simulink model "main"  (R2022a)
settings: Solver=FixedStepDiscrete  StartTime=0.0  StopTime=Inf  FixedStep=(50e-6)-(sim_en*4.995e-5)  RelTol=1e-3  EnableMultiTasking=on
model workspace (MAT data in the model file):
  Param : Simulink.Parameter (value not decoded)
  ac_ok : Simulink.Signal (value not decoded)
  ac_ok_120 : Simulink.Signal (value not decoded)
  bulk_voltage : Simulink.Signal (value not decoded)
  burstduty_integ_max : Simulink.Signal (value not decoded)
  burstduty_integ_min : Simulink.Signal (value not decoded)
  burstduty_ki : Simulink.Signal (value not decoded)
  burstduty_kp : Simulink.Signal (value not decoded)
  calib_ok : Simulink.Signal (value not decoded)
  can_addr1 : Simulink.Signal (value not decoded)
  can_addr2 : Simulink.Signal (value not decoded)
  can_addr3 : Simulink.Signal (value not decoded)
  can_addr4 : Simulink.Signal (value not decoded)
  can_data_rx : Simulink.Signal (value not decoded)
  can_data_tx : Simulink.Signal (value not decoded)
  can_timeout_120 : Simulink.Signal (value not decoded)
  chksum_scircv : Simulink.Signal (value not decoded)
  clllc_en_120 : Simulink.Signal (value not decoded)
  clllc_fault_120 : Simulink.Signal (value not decoded)
  clllc_ok_120 : Simulink.Signal (value not decoded)
  cmpss1h : Simulink.Signal (value not decoded)
  cmpss1l : Simulink.Signal (value not decoded)
  cmpss2h : Simulink.Signal (value not decoded)
  cmpss2l : Simulink.Signal (value not decoded)
  cmpss3h : Simulink.Signal (value not decoded)
  cmpss3l : Simulink.Signal (value not decoded)
  cmpss4h : Simulink.Signal (value not decoded)
  cmpss4l : Simulink.Signal (value not decoded)
  cmpss5h : Simulink.Signal (value not decoded)
  cmpss5l : Simulink.Signal (value not decoded)
  cmpss6h : Simulink.Signal (value not decoded)
  cmpss6l : Simulink.Signal (value not decoded)
  cmpss7h : Simulink.Signal (value not decoded)
  cmpss7l : Simulink.Signal (value not decoded)
  cmpss8h : Simulink.Signal (value not decoded)
  cmpss8l : Simulink.Signal (value not decoded)
  cnt_idle : Simulink.Signal (value not decoded)
  cnt_orps : Simulink.Signal (value not decoded)
  cnt_scircv : Simulink.Signal (value not decoded)
  cnt_scixmt : Simulink.Signal (value not decoded)
  cnt_scixmt_func : Simulink.Signal (value not decoded)
  cnt_temp_mux : Simulink.Signal (value not decoded)
  cnt_vdroop : Simulink.Signal (value not decoded)
  config_ok : Simulink.Signal (value not decoded)
  control_en : Simulink.Signal (value not decoded)
  cp_ready_120 : Simulink.Signal (value not decoded)
  d2d_en : Simulink.Signal (value not decoded)
  dchg_off : Simulink.Signal (value not decoded)
  debug_dacb : Simulink.Signal (value not decoded)
  debug_dacc : Simulink.Signal (value not decoded)
  debug_msg1 : Simulink.Signal (value not decoded)
  debug_msg2 : Simulink.Signal (value not decoded)
  debug_msg3 : Simulink.Signal (value not decoded)
  debug_msg4 : Simulink.Signal (value not decoded)
  debug_msg5 : Simulink.Signal (value not decoded)
  debug_msg6 : Simulink.Signal (value not decoded)
  dir_v2g : Simulink.Signal (value not decoded)
  eoss_llc1 : Simulink.Signal (value not decoded)
  eoss_llc2 : Simulink.Signal (value not decoded)
  eoss_orps : Simulink.Signal (value not decoded)
  fault_ocp : Simulink.Signal (value not decoded)
  fault_otp : Simulink.Signal (value not decoded)
  fault_ovp : Simulink.Signal (value not decoded)
  fut_en : Simulink.Signal (value not decoded)
  fwd_en_120 : Simulink.Signal (value not decoded)
  gain_llc1_sec_idc : Simulink.Signal (value not decoded)
  gain_llc1_temp_sr : Simulink.Signal (value not decoded)
  gain_llc2_sec_idc : Simulink.Signal (value not decoded)
  gain_vbat : Simulink.Signal (value not decoded)
  gain_vbulk : Simulink.Signal (value not decoded)
  gain_vout : Simulink.Signal (value not decoded)
  input_current_phasea : Simulink.Signal (value not decoded)
  input_current_phaseb : Simulink.Signal (value not decoded)
  input_current_phasec : Simulink.Signal (value not decoded)
  input_freq : Simulink.Signal (value not decoded)
  input_power : Simulink.Signal (value not decoded)
  input_voltage_phasea : Simulink.Signal (value not decoded)
  input_voltage_phaseb : Simulink.Signal (value not decoded)
  input_voltage_phasec : Simulink.Signal (value not decoded)
  ishare_arbiter : Simulink.Signal (value not decoded)
  ishare_thresh : Simulink.Signal (value not decoded)
  led_g : Simulink.Signal (value not decoded)
  led_r : Simulink.Signal (value not decoded)
  led_y : Simulink.Signal (value not decoded)
  llc1_burst_integ : Simulink.Signal (value not decoded)
  llc1_burstduty_buffer : Simulink.Signal (value not decoded)
  llc1_pfm_error : Simulink.Signal (value not decoded)
  llc1_pfm_integ : Simulink.Signal (value not decoded)
  llc1_pfm_prop : Simulink.Signal (value not decoded)
  llc1_pri_idc : Simulink.Signal (value not decoded)
  llc1_ps_buffer : Simulink.Signal (value not decoded)
  llc1_pspwm_error : Simulink.Signal (value not decoded)
  llc1_pspwm_integ : Simulink.Signal (value not decoded)
  llc1_pspwm_prop : Simulink.Signal (value not decoded)
  llc1_sec_idc : Simulink.Signal (value not decoded)
  llc1_temp_sr : Simulink.Signal (value not decoded)
  llc1_ts_tbctr_buffer : Simulink.Signal (value not decoded)
  llc2_burst_integ : Simulink.Signal (value not decoded)
  llc2_burstduty_buffer : Simulink.Signal (value not decoded)
  llc2_en : Simulink.Signal (value not decoded)
  llc2_en_buffer : Simulink.Signal (value not decoded)
  llc2_pfm_error : Simulink.Signal (value not decoded)
  llc2_pfm_integ : Simulink.Signal (value not decoded)
  llc2_pfm_prop : Simulink.Signal (value not decoded)
  llc2_pri_idc : Simulink.Signal (value not decoded)
  llc2_ps_buffer : Simulink.Signal (value not decoded)
  llc2_pspwm_error : Simulink.Signal (value not decoded)
  llc2_pspwm_integ : Simulink.Signal (value not decoded)
  llc2_pspwm_prop : Simulink.Signal (value not decoded)
  llc2_sec_idc : Simulink.Signal (value not decoded)
  llc2_temp_sr : Simulink.Signal (value not decoded)
  llc2_ts_tbctr_buffer : Simulink.Signal (value not decoded)
  loop_adcint : Simulink.Signal (value not decoded)
  loop_control : Simulink.Signal (value not decoded)
  loop_idle : Simulink.Signal (value not decoded)
  mid_bulk_voltage : Simulink.Signal (value not decoded)
  mode_120 : Simulink.Signal (value not decoded)
  mode_cc_cv : Simulink.Signal (value not decoded)
  myParam : mpt.Parameter (value not decoded)
  obc_ok_120 : Simulink.Signal (value not decoded)
  offset_llc1_sec_idc : Simulink.Signal (value not decoded)
  offset_llc1_temp_sr : Simulink.Signal (value not decoded)
  offset_llc2_sec_idc : Simulink.Signal (value not decoded)
  offset_vbat : Simulink.Signal (value not decoded)
  offset_vbulk : Simulink.Signal (value not decoded)
  offset_vout : Simulink.Signal (value not decoded)
  openloop_en : Simulink.Signal (value not decoded)
  openloop_fault_en : Simulink.Signal (value not decoded)
  ot_fault_120 : Simulink.Signal (value not decoded)
  pfc_en : Simulink.Signal (value not decoded)
  pfc_en_120 : Simulink.Signal (value not decoded)
  pfc_fw_revision : Simulink.Signal (value not decoded)
  pfc_fw_revision_bootloader : Simulink.Signal (value not decoded)
  pfc_fw_revision_debug : Simulink.Signal (value not decoded)
  pfc_ok : Simulink.Signal (value not decoded)
  pfc_ok_120 : Simulink.Signal (value not decoded)
  pfm_a0 : Simulink.Signal (value not decoded)
  pfm_a1 : Simulink.Signal (value not decoded)
  pfm_integ_max : Simulink.Signal (value not decoded)
  pfm_integ_min : Simulink.Signal (value not decoded)
  pfm_ki : Simulink.Signal (value not decoded)
  pfm_kp : Simulink.Signal (value not decoded)
  pri_fut_en : Simulink.Signal (value not decoded)
  pri_fut_en_buffer : Simulink.Signal (value not decoded)
  pri_halfbridge_en : Simulink.Signal (value not decoded)
  pri_halfbridge_en_buffer : Simulink.Signal (value not decoded)
  pspwm_integ_max : Simulink.Signal (value not decoded)
  pspwm_integ_min : Simulink.Signal (value not decoded)
  pspwm_ki : Simulink.Signal (value not decoded)
  pspwm_kp : Simulink.Signal (value not decoded)
  ref_idclink_max : Simulink.Signal (value not decoded)
  ref_iout : Simulink.Signal (value not decoded)
  ref_iout_calib : Simulink.Signal (value not decoded)
  ref_iout_llc1 : Simulink.Signal (value not decoded)
  ref_iout_llc1_calib : Simulink.Signal (value not decoded)
  ref_iout_llc2 : Simulink.Signal (value not decoded)
  ref_iout_llc2_calib : Simulink.Signal (value not decoded)
  ref_pout : Simulink.Signal (value not decoded)
  ref_ss_llc1 : Simulink.Signal (value not decoded)
  ref_ss_llc2 : Simulink.Signal (value not decoded)
  ref_ss_orps : Simulink.Signal (value not decoded)
  ref_vbat : Simulink.Signal (value not decoded)
  ref_vbat_calib : Simulink.Signal (value not decoded)
  ref_vbulk : Simulink.Signal (value not decoded)
  ref_vbulk_calib : Simulink.Signal (value not decoded)
  ref_vbulk_llc1_calib : Simulink.Signal (value not decoded)
  ref_vbulk_llc2_calib : Simulink.Signal (value not decoded)
  ref_vout : Simulink.Signal (value not decoded)
  ref_vout_calib : Simulink.Signal (value not decoded)
  relay_en : Simulink.Signal (value not decoded)
  reset_flag : Simulink.Signal (value not decoded)
  rev_en_120 : Simulink.Signal (value not decoded)
  runtime_control : Simulink.Signal (value not decoded)
  runtime_idle : Simulink.Signal (value not decoded)
  scircv_buffer : Simulink.Signal (value not decoded)
  scircv_buffer_tmp : Simulink.Signal (value not decoded)
  scircv_buffer_tmp_idx0 : Simulink.Signal (value not decoded)
  scircv_chksum : Simulink.Signal (value not decoded)
  scircv_chksum_ok : Simulink.Signal (value not decoded)
  scircv_parse_ok : Simulink.Signal (value not decoded)
  scixmt_buffer : Simulink.Signal (value not decoded)
  scixmt_chksum : Simulink.Signal (value not decoded)
  scixmt_func : Simulink.Signal (value not decoded)
  scixmt_word0_lsb : Simulink.Signal (value not decoded)
  scixmt_word0_msb : Simulink.Signal (value not decoded)
  scixmt_word1_lsb : Simulink.Signal (value not decoded)
  scixmt_word1_msb : Simulink.Signal (value not decoded)
  scixmt_word2_lsb : Simulink.Signal (value not decoded)
  scixmt_word2_msb : Simulink.Signal (value not decoded)
  scixmt_wr : Simulink.Signal (value not decoded)
  ss_step : Simulink.Signal (value not decoded)
  state_calib : Simulink.Signal (value not decoded)
  state_control : Simulink.Signal (value not decoded)
  state_hkeep : Simulink.Signal (value not decoded)
  status_cmpss : Simulink.Signal (value not decoded)
  status_control : Simulink.Signal (value not decoded)
  status_digin : Simulink.Signal (value not decoded)
  status_digout : Simulink.Signal (value not decoded)
  status_fault : Simulink.Signal (value not decoded)
  status_input : Simulink.Signal (value not decoded)
  status_pfc : Simulink.Signal (value not decoded)
  temp_inlet : Simulink.Signal (value not decoded)
  temp_llc1_fet_hs : Simulink.Signal (value not decoded)
  temp_llc2_fet_hs : Simulink.Signal (value not decoded)
  temp_mux : Simulink.Signal (value not decoded)
  temp_mux_s0 : Simulink.Signal (value not decoded)
  temp_mux_s1 : Simulink.Signal (value not decoded)
  temp_mux_s2 : Simulink.Signal (value not decoded)
  temp_outlet : Simulink.Signal (value not decoded)
  temp_pfc_fet_hsa : Simulink.Signal (value not decoded)
  temp_pfc_fet_hsb : Simulink.Signal (value not decoded)
  temp_pfc_fet_hsc : Simulink.Signal (value not decoded)
  temp_pfc_fet_lsa : Simulink.Signal (value not decoded)
  temp_pfc_fet_lsb : Simulink.Signal (value not decoded)
  temp_pfc_fet_lsc : Simulink.Signal (value not decoded)
  test_mode : Simulink.Signal (value not decoded)
  tfcv_cc : Simulink.Signal (value not decoded)
  tfcv_cc_llc2 : Simulink.Signal (value not decoded)
  tfcv_cv : Simulink.Signal (value not decoded)
  tfcv_sr_en : Simulink.Signal (value not decoded)
  tfv_assert_llc1_pri_idc : Simulink.Signal (value not decoded)
  tfv_assert_llc1_sec_idc : Simulink.Signal (value not decoded)
  tfv_assert_llc1_temp_sr : Simulink.Signal (value not decoded)
  tfv_assert_llc2_pri_idc : Simulink.Signal (value not decoded)
  tfv_assert_llc2_sec_idc : Simulink.Signal (value not decoded)
  tfv_assert_llc2_temp_sr : Simulink.Signal (value not decoded)
  tfv_assert_temp_outlet : Simulink.Signal (value not decoded)
  tfv_assert_vaux_uv : Simulink.Signal (value not decoded)
  tfv_assert_vbat : Simulink.Signal (value not decoded)
  tfv_assert_vbulk : Simulink.Signal (value not decoded)
  tfv_assert_vout : Simulink.Signal (value not decoded)
  tfv_cnt_tz : Simulink.Signal (value not decoded)
  tfv_deassert_llc1_pri_idc : Simulink.Signal (value not decoded)
  tfv_deassert_llc1_sec_idc : Simulink.Signal (value not decoded)
  tfv_deassert_llc1_temp_sr : Simulink.Signal (value not decoded)
  tfv_deassert_llc2_pri_idc : Simulink.Signal (value not decoded)
  tfv_deassert_llc2_sec_idc : Simulink.Signal (value not decoded)
  tfv_deassert_llc2_temp_sr : Simulink.Signal (value not decoded)
  tfv_deassert_temp_outlet : Simulink.Signal (value not decoded)
  tfv_deassert_vaux_uv : Simulink.Signal (value not decoded)
  tfv_deassert_vbat : Simulink.Signal (value not decoded)
  tfv_deassert_vbulk : Simulink.Signal (value not decoded)
  tfv_deassert_vout : Simulink.Signal (value not decoded)
  tfv_llc1_pri_idc : Simulink.Signal (value not decoded)
  tfv_llc1_sec_idc : Simulink.Signal (value not decoded)
  tfv_llc1_temp_sr : Simulink.Signal (value not decoded)
  tfv_llc2_pri_idc : Simulink.Signal (value not decoded)
  tfv_llc2_sec_idc : Simulink.Signal (value not decoded)
  tfv_llc2_temp_sr : Simulink.Signal (value not decoded)
  tfv_temp_outlet : Simulink.Signal (value not decoded)
  tfv_vaux_uv : Simulink.Signal (value not decoded)
  tfv_vbat : Simulink.Signal (value not decoded)
  tfv_vbulk : Simulink.Signal (value not decoded)
  tfv_vout : Simulink.Signal (value not decoded)
  timer_1ms : Simulink.Signal (value not decoded)
  tz : Simulink.Signal (value not decoded)
  valve_en : Simulink.Signal (value not decoded)
  vaux : Simulink.Signal (value not decoded)
  vbat : Simulink.Signal (value not decoded)
  vbulk : Simulink.Signal (value not decoded)
  vout : Simulink.Signal (value not decoded)
undefined symbols (not defined in the file or in its folder): CAN_O_INT, CANA_BASE, Down, GPTRIP1SEL, GPTRIP2SEL, TZ1, TZ2, Up
libraries: hdlsllib x159, simulink x94, c2802xlib x32, c2837xDlib x19, c2807xlib x16, c280xlib x13, canmsglib x8, idelinklib_common x2, c2000lib x1, c281xlib x1
(part 16 of 20)

== system main/Task_Manager/init/codegen/init/tztl_clb/clb ==
  note: // Enabling EPWM1 to enable CLB1
      | SysCtl_enablePeripheral(SYSCTL_PERIPH_CLK_EPWM1);
      | CLB_enableCLB(CLB1_BASE);
      | initTILE0(CLB1_BASE);
      |
      | // Enabling EPWM2 to enable CLB2
      | SysCtl_enablePeripheral(SYSCTL_PERIPH_CLK_EPWM1);
      | CLB_enableCLB(CLB2_BASE);
      | initTILE1(CLB2_BASE);
      |
      |
      |
      | // Select Global input instead of local input for all CLB IN
      | CLB_configLocalInputMux(CLB1_BASE, CLB_IN0, CLB_LOCAL_IN_MUX_GLOBAL_IN);
      | CLB_configLocalInputMux(CLB1_BASE, CLB_IN1, CLB_LOCAL_IN_MUX_GLOBAL_IN);
      | CLB_configLocalInputMux(CLB1_BASE, CLB_IN2, CLB_LOCAL_IN_MUX_GLOBAL_IN);
      | CLB_configLocalInputMux(CLB1_BASE, CLB_IN3, CLB_LOCAL_IN_MUX_GLOBAL_IN);
      | CLB_configLocalInputMux(CLB1_BASE, CLB_IN4, CLB_LOCAL_IN_MUX_GLOBAL_IN);
      | CLB_configLocalInputMux(CLB1_BASE, CLB_IN5, CLB_LOCAL_IN_MUX_GLOBAL_IN);
      | CLB_configLocalInputMux(CLB1_BASE, CLB_IN6, CLB_LOCAL_IN_MUX_GLOBAL_IN);
      | CLB_configLocalInputMux(CLB1_BASE, CLB_IN7, CLB_LOCAL_IN_MUX_GLOBAL_IN);
      |
      | CLB_configLocalInputMux(CLB2_BASE, CLB_IN0, CLB_LOCAL_IN_MUX_GLOBAL_IN);
      | CLB_configLocalInputMux(CLB2_BASE, CLB_IN1, CLB_LOCAL_IN_MUX_GLOBAL_IN);
      | CLB_configLocalInputMux(CLB2_BASE, CLB_IN2, CLB_LOCAL_IN_MUX_GLOBAL_IN);
      | CLB_configLocalInputMux(CLB2_BASE, CLB_IN3, CLB_LOCAL_IN_MUX_GLOBAL_IN);
      | CLB_configLocalInputMux(CLB2_BASE, CLB_IN4, CLB_LOCAL_IN_MUX_GLOBAL_IN);
      | CLB_configLocalInputMux(CLB2_BASE, CLB_IN5, CLB_LOCAL_IN_MUX_GLOBAL_IN);
      | CLB_configLocalInputMux(CLB2_BASE, CLB_IN6, CLB_LOCAL_IN_MUX_GLOBAL_IN);
      | CLB_configLocalInputMux(CLB2_BASE, CLB_IN7, CLB_LOCAL_IN_MUX_GLOBAL_IN);
      |
      |
      | // Select AUXSIG for CLBx, IN0/1/2
      | CLB_configGlobalInputMux(CLB1_BASE, CLB_IN0, CLB_GLOBAL_IN_MUX_CLB_AUXSIG0);
      | CLB_configGlobalInputMux(CLB1_BASE, CLB_IN1, CLB_GLOBAL_IN_MUX_CLB_AUXSIG1);
      | CLB_configGlobalInputMux(CLB1_BASE, CLB_IN2, CLB_GLOBAL_IN_MUX_EPWM1_CTR_PRD);
      | CLB_configGlobalInputMux(CLB2_BASE, CLB_IN0, CLB_GLOBAL_IN_MUX_CLB_AUXSIG2);
      | CLB_configGlobalInputMux(CLB2_BASE, CLB_IN1, CLB_GLOBAL_IN_MUX_CLB_AUXSIG3);
      | CLB_configGlobalInputMux(CLB2_BASE, CLB_IN2, CLB_GLOBAL_IN_MUX_EPWM1_CTR_ZERO);
      |
      |
      | // Unused inputs below
      | CLB_configGlobalInputMux(CLB1_BASE, CLB_IN3, CLB_GLOBAL_IN_MUX_EPWM1A);
      | CLB_configGlobalInputMux(CLB1_BASE, CLB_IN4, CLB_GLOBAL_IN_MUX_EPWM1A);
      | CLB_configGlobalInputMux(CLB1_BASE, CLB_IN5, CLB_GLOBAL_IN_MUX_EPWM1A);
      | CLB_configGlobalInputMux(CLB1_BASE, CLB_IN6, CLB_GLOBAL_IN_MUX_EPWM1A);
      | CLB_configGlobalInputMux(CLB1_BASE, CLB_IN7, CLB_GLOBAL_IN_MUX_EPWM1A);
      | CLB_configGlobalInputMux(CLB2_BASE, CLB_IN3, CLB_GLOBAL_IN_MUX_EPWM1A);
      | CLB_configGlobalInputMux(CLB2_BASE, CLB_IN4, CLB_GLOBAL_IN_MUX_EPWM1A);
      | CLB_configGlobalInputMux(CLB2_BASE, CLB_IN5, CLB_GLOBAL_IN_MUX_EPWM1A);
      | CLB_configGlobalInputMux(CLB2_BASE, CLB_IN6, CLB_GLOBAL_IN_MUX_EPWM1A);
      | CLB_configGlobalInputMux(CLB2_BASE, CLB_IN7, CLB_GLOBAL_IN_MUX_EPWM1A);
      |
      |
      | // Set CLB_IN to mux external
      | CLB_configGPInputMux(CLB1_BASE, CLB_IN0, CLB_GP_IN_MUX_EXTERNAL);
      | CLB_configGPInputMux(CLB1_BASE, CLB_IN1, CLB_GP_IN_MUX_EXTERNAL);
      | CLB_configGPInputMux(CLB1_BASE, CLB_IN2, CLB_GP_IN_MUX_EXTERNAL);
      | CLB_configGPInputMux(CLB2_BASE, CLB_IN0, CLB_GP_IN_MUX_EXTERNAL);
      | CLB_configGPInputMux(CLB2_BASE, CLB_IN1, CLB_GP_IN_MUX_EXTERNAL);
      | CLB_configGPInputMux(CLB2_BASE, CLB_IN2, CLB_GP_IN_MUX_EXTERNAL);
      |
      |
      | // Set unused inputs to GP register
      | CLB_configGPInputMux(CLB1_BASE, CLB_IN3, CLB_GP_IN_MUX_GP_REG);
      | CLB_configGPInputMux(CLB1_BASE, CLB_IN4, CLB_GP_IN_MUX_GP_REG);
      | CLB_configGPInputMux(CLB1_BASE, CLB_IN5, CLB_GP_IN_MUX_GP_REG);
      | CLB_configGPInputMux(CLB1_BASE, CLB_IN6, CLB_GP_IN_MUX_GP_REG);
      | CLB_configGPInputMux(CLB1_BASE, CLB_IN7, CLB_GP_IN_MUX_GP_REG);
      | CLB_configGPInputMux(CLB2_BASE, CLB_IN3, CLB_GP_IN_MUX_GP_REG);
      | CLB_configGPInputMux(CLB2_BASE, CLB_IN4, CLB_GP_IN_MUX_GP_REG);
      | CLB_configGPInputMux(CLB2_BASE, CLB_IN5, CLB_GP_IN_MUX_GP_REG);
      | CLB_configGPInputMux(CLB2_BASE, CLB_IN6, CLB_GP_IN_MUX_GP_REG);
      | CLB_configGPInputMux(CLB2_BASE, CLB_IN7, CLB_GP_IN_MUX_GP_REG);
      |
      |
      | // Configure CLB-XBAR AUXSIG
      | XBAR_setCLBMuxConfig(XBAR_AUXSIG0, XBAR_CLB_MUX08_CMPSS5_CTRIPH);
      | XBAR_enableCLBMux(XBAR_AUXSIG0, XBAR_MUX08);
      | XBAR_setCLBMuxConfig(XBAR_AUXSIG1, XBAR_CLB_MUX09_CMPSS5_CTRIPL);
      | XBAR_enableCLBMux(XBAR_AUXSIG1, XBAR_MUX09);
      | XBAR_setCLBMuxConfig(XBAR_AUXSIG2, XBAR_CLB_MUX10_CMPSS6_CTRIPH);
      | XBAR_enableCLBMux(XBAR_AUXSIG2, XBAR_MUX10);
      | XBAR_setCLBMuxConfig(XBAR_AUXSIG3, XBAR_CLB_MUX11_CMPSS6_CTRIPL);
      | XBAR_enableCLBMux(XBAR_AUXSIG3, XBAR_MUX11);
      |
      |
      |
      | // Configure ePWM XBAR
      | XBAR_setEPWMMuxConfig(XBAR_TRIP9, XBAR_EPWM_MUX01_CLB1_OUT4);
      | XBAR_enableEPWMMux(XBAR_TRIP9, XBAR_MUX01);
      | XBAR_setEPWMMuxConfig(XBAR_TRIP10, XBAR_EPWM_MUX05_CLB2_OUT4);
      | XBAR_enableEPWMMux(XBAR_TRIP10, XBAR_MUX05);
  function : TriggerPort  TriggerType=function-call  VariantControl=Variant
  System Initialize : Subsystem  mask(System Initialize){ShowInLibBrowser=0}
      mask prompts: ShowInLibBrowser "Simulink:masks:CustCodeMaskParam1_MP"
      settings: CopyFcn=cccopyfcn(gcb)  OpenFcn=ccopenfcn('System Initialize Function')
      mask Help: eval('feval(''rtwprivate'',''rtwhelpview'',''rtw_sys_initialize_block'')');
      mask Display: disp('System\nInitialize');

== system main/Task_Manager/init/codegen/init/tztl_clb/tzctl ==
  note: //TZCTL configures TZ action of a DCxEVTy event
      | //0b00=HI-Z, 0b01=HI, 0b10=LO, 0b11=DN
      | EALLOW;
      |
      | //LLC1_PRI_PS
      | EPwm1Regs.TZCTL.bit.DCAEVT1 = 0b11; //Do nothing
      | EPwm1Regs.TZCTL.bit.DCAEVT2 = 0b11; //Do nothing
      | EPwm1Regs.TZCTL.bit.DCBEVT1 = 0b11; //Do nothing
      | EPwm1Regs.TZCTL.bit.DCBEVT2 = 0b11; //Do nothing
      |
      | //LLC1_PRI_STD
      | EPwm2Regs.TZCTL.bit.DCAEVT1 = 0b11; //Do nothing
      | EPwm2Regs.TZCTL.bit.DCAEVT2 = 0b11; //Do nothing
      | EPwm2Regs.TZCTL.bit.DCBEVT1 = 0b11; //Do nothing
      | EPwm2Regs.TZCTL.bit.DCBEVT2 = 0b11; //Do nothing
      |
      | //LLC1_SEC_PS
      | EPwm7Regs.TZCTL.bit.DCAEVT1 = 0b10; //LO
      | EPwm7Regs.TZCTL.bit.DCAEVT2 = 0b01; //HI
      | EPwm7Regs.TZCTL.bit.DCBEVT1 = 0b10; //LO
      | EPwm7Regs.TZCTL.bit.DCBEVT2 = 0b01; //HI
      |
      | //LLC1_SEC_STD
      | EPwm8Regs.TZCTL.bit.DCAEVT1 = 0b10; //LO
      | EPwm8Regs.TZCTL.bit.DCAEVT2 = 0b01; //HI
      | EPwm8Regs.TZCTL.bit.DCBEVT1 = 0b10; //LO
      | EPwm8Regs.TZCTL.bit.DCBEVT2 = 0b01; //HI
      |
      | EDIS;
  function : TriggerPort  TriggerType=function-call  VariantControl=Variant
  System Initialize : Subsystem  mask(System Initialize){ShowInLibBrowser=0}
      mask prompts: ShowInLibBrowser "Simulink:masks:CustCodeMaskParam1_MP"
      settings: CopyFcn=cccopyfcn(gcb)  OpenFcn=ccopenfcn('System Initialize Function')
      mask Help: eval('feval(''rtwprivate'',''rtwhelpview'',''rtw_sys_initialize_block'')');
      mask Display: disp('System\nInitialize');

== system main/interrupt_adca/burst_control/burst/disPulse/Variant Subsystem/codegen/g2v_prifullbridge ==
  note: EPwm1Regs.AQCSFRC.bit.CSFA = 0b1; //force low
      | EPwm1Regs.AQCSFRC.bit.CSFB = 0b1; //force low
      | EPwm2Regs.AQCSFRC.bit.CSFA = 0b1; //force low
      | EPwm2Regs.AQCSFRC.bit.CSFB = 0b1; //force low
      |
      | EPwm7Regs.AQCSFRC.bit.CSFA = 0b1; //force low
      | EPwm7Regs.AQCSFRC.bit.CSFB = 0b1; //force low
      | EPwm8Regs.AQCSFRC.bit.CSFA = 0b1; //force low
      | EPwm8Regs.AQCSFRC.bit.CSFB = 0b1; //force low
  Action Port : ActionPort  ActionPortLabel=if((u1==0))
  System Outputs1 : Subsystem  mask(System Outputs){ShowInLibBrowser=0}
      mask prompts: ShowInLibBrowser "Simulink:masks:CustCodeMaskParam1_MP"
      settings: CopyFcn=cccopyfcn(gcb)  OpenFcn=ccopenfcn('System Outputs Function')
      mask Help: eval('feval(''rtwprivate'',''rtwhelpview'',''rtw_sys_outputs_block'')');
      mask DialogControl ShowInLibBrowser Prompt: Mask Parameter 1:
      mask Display: disp('System\nOutputs');

== system main/interrupt_adca/burst_control/burst/disPulse/Variant Subsystem/codegen/v2g_prifullbridge ==
  note: EPwm1Regs.AQCSFRC.bit.CSFA = 0b1; //force low
      | EPwm1Regs.AQCSFRC.bit.CSFB = 0b1; //force low
      | EPwm2Regs.AQCSFRC.bit.CSFA = 0b1; //force low
      | EPwm2Regs.AQCSFRC.bit.CSFB = 0b1; //force low
      | EPwm7Regs.AQCSFRC.bit.CSFA = 0b1; //force low
      | EPwm7Regs.AQCSFRC.bit.CSFB = 0b1; //force low
      | EPwm8Regs.AQCSFRC.bit.CSFA = 0b1; //force low
      | EPwm8Regs.AQCSFRC.bit.CSFB = 0b1; //force low
  Action Port : ActionPort  ActionPortLabel=elseif((u1==1))
  System Outputs1 : Subsystem  mask(System Outputs){ShowInLibBrowser=0}
      mask prompts: ShowInLibBrowser "Simulink:masks:CustCodeMaskParam1_MP"
      settings: CopyFcn=cccopyfcn(gcb)  OpenFcn=ccopenfcn('System Outputs Function')
      mask Help: eval('feval(''rtwprivate'',''rtwhelpview'',''rtw_sys_outputs_block'')');
      mask DialogControl ShowInLibBrowser Prompt: Mask Parameter 1:
      mask Display: disp('System\nOutputs');

== system main/interrupt_adca/burst_control/burst/disPulse/Variant Subsystem/sim/g2v_prifullbridge ==
  note: EPwm1Regs.AQCSFRC.bit.CSFA = 0b1; //force low
      | EPwm1Regs.AQCSFRC.bit.CSFB = 0b1; //force low
      | EPwm2Regs.AQCSFRC.bit.CSFA = 0b1; //force low
      | EPwm2Regs.AQCSFRC.bit.CSFB = 0b1; //force low
      | EPwm7Regs.AQCSFRC.bit.CSFA = 0b0; //force disable
      | EPwm7Regs.AQCSFRC.bit.CSFB = 0b0; //force disable
      | EPwm8Regs.AQCSFRC.bit.CSFA = 0b0; //force disable
      | EPwm8Regs.AQCSFRC.bit.CSFB = 0b0; //force disable
  note: LLC1 SEC
  note: LLC1 PRI
  Action Port : ActionPort
  Constant{,1,4..5} (4 alike) : Constant  OutDataTypeStr=boolean
  Constant{2..3,6..7} (4 alike) : Constant  Value=0  OutDataTypeStr=boolean
  Data Store Write : DataStoreWrite  DataStoreName=epwm1_aqcsfrc_csfa  IndexOptions=Index vector (dialog)  Indices=1  OutputSizes=1
  Data Store Write1 : DataStoreWrite  DataStoreName=epwm1_aqcsfrc_csfb  IndexOptions=Index vector (dialog)  Indices=1  OutputSizes=1
  Data Store Write2 : DataStoreWrite  DataStoreName=epwm7_aqcsfrc_csfa  IndexOptions=Index vector (dialog)  Indices=1  OutputSizes=1
  Data Store Write3 : DataStoreWrite  DataStoreName=epwm7_aqcsfrc_csfb  IndexOptions=Index vector (dialog)  Indices=1  OutputSizes=1
  Data Store Write4 : DataStoreWrite  DataStoreName=epwm2_aqcsfrc_csfa  IndexOptions=Index vector (dialog)  Indices=1  OutputSizes=1
  Data Store Write5 : DataStoreWrite  DataStoreName=epwm2_aqcsfrc_csfb  IndexOptions=Index vector (dialog)  Indices=1  OutputSizes=1
  Data Store Write6 : DataStoreWrite  DataStoreName=epwm8_aqcsfrc_csfa  IndexOptions=Index vector (dialog)  Indices=1  OutputSizes=1
  Data Store Write7 : DataStoreWrite  DataStoreName=epwm8_aqcsfrc_csfb  IndexOptions=Index vector (dialog)  Indices=1  OutputSizes=1
  wires:
  Constant3/1 -> Data Store Write3/1
  Constant2/1 -> Data Store Write2/1
  Constant6/1 -> Data Store Write6/1
  Constant/1 -> Data Store Write/1
  Constant4/1 -> Data Store Write4/1
  Constant1/1 -> Data Store Write1/1
  Constant5/1 -> Data Store Write5/1
  Constant7/1 -> Data Store Write7/1

== system main/interrupt_adca/burst_control/burst/disPulse/Variant Subsystem/sim/v2g_prifullbridge ==
  note: EPwm1Regs.AQCSFRC.bit.CSFA = 0b0; //force disabled
      | EPwm1Regs.AQCSFRC.bit.CSFB = 0b0; //force disabled
      | EPwm2Regs.AQCSFRC.bit.CSFA = 0b0; //force disabled
      | EPwm2Regs.AQCSFRC.bit.CSFB = 0b0; //force disabled
      | EPwm7Regs.AQCSFRC.bit.CSFA = 0b1; //force low
      | EPwm7Regs.AQCSFRC.bit.CSFB = 0b1; //force low
      | EPwm8Regs.AQCSFRC.bit.CSFA = 0b1; //force low
      | EPwm8Regs.AQCSFRC.bit.CSFB = 0b1; //force low
  note: LLC1 SEC
  note: LLC1 PRI
  Action Port : ActionPort
  Constant{,1,4..5} (4 alike) : Constant  Value=0  OutDataTypeStr=boolean
  Constant{2..3,6..7} (4 alike) : Constant  OutDataTypeStr=boolean
  Data Store Write : DataStoreWrite  DataStoreName=epwm1_aqcsfrc_csfa  IndexOptions=Index vector (dialog)  Indices=1  OutputSizes=1
  Data Store Write1 : DataStoreWrite  DataStoreName=epwm1_aqcsfrc_csfb  IndexOptions=Index vector (dialog)  Indices=1  OutputSizes=1
  Data Store Write2 : DataStoreWrite  DataStoreName=epwm7_aqcsfrc_csfa  IndexOptions=Index vector (dialog)  Indices=1  OutputSizes=1
  Data Store Write3 : DataStoreWrite  DataStoreName=epwm7_aqcsfrc_csfb  IndexOptions=Index vector (dialog)  Indices=1  OutputSizes=1
  Data Store Write4 : DataStoreWrite  DataStoreName=epwm2_aqcsfrc_csfa  IndexOptions=Index vector (dialog)  Indices=1  OutputSizes=1
  Data Store Write5 : DataStoreWrite  DataStoreName=epwm2_aqcsfrc_csfb  IndexOptions=Index vector (dialog)  Indices=1  OutputSizes=1
  Data Store Write6 : DataStoreWrite  DataStoreName=epwm8_aqcsfrc_csfa  IndexOptions=Index vector (dialog)  Indices=1  OutputSizes=1
  Data Store Write7 : DataStoreWrite  DataStoreName=epwm8_aqcsfrc_csfb  IndexOptions=Index vector (dialog)  Indices=1  OutputSizes=1
  wires:
  Constant6/1 -> Data Store Write6/1
  Constant2/1 -> Data Store Write2/1
  Constant3/1 -> Data Store Write3/1
  Constant5/1 -> Data Store Write5/1
  Constant1/1 -> Data Store Write1/1
  Constant4/1 -> Data Store Write4/1
  Constant/1 -> Data Store Write/1
  Constant7/1 -> Data Store Write7/1

== system main/interrupt_adca/burst_control/burst/disPwm/disPwm/codegen/System Outputs1 ==

== system main/interrupt_adca/burst_control/burst/enPulse/enPwm/codegen/System Outputs ==

== system main/Control_State_Machine/control/configSr/configXbarEpwmtrip/codegen/g2v_prifullbridge/clb/System Outputs1 ==

== system main/Control_State_Machine/control/configSr/configXbarEpwmtrip/codegen/g2v_prifullbridge/tzctl/System Outputs ==

== system main/Control_State_Machine/control/configSr/configXbarEpwmtrip/codegen/v2g_prifullbridge/clb/System Outputs3 ==

== system main/Control_State_Machine/control/configSr/configXbarEpwmtrip/codegen/v2g_prifullbridge/tzctl/System Outputs1 ==

== system main/Task_Manager/Tmr_20mS/codegen/Task_20mS/Rx_Handler/ProcessMB10/Mode_Cmd ==
  Input : Inport
  Action Port : ActionPort  ActionPortLabel=if(u1 == 1)
  Data Store Write1 : DataStoreWrite  DataStoreName=u8ModeCmd  IndexOptions=Index vector (dialog)  Indices=1  OutputSizes=1
  wires:
  Input/1 -> Data Store Write1/1

== system main/Task_Manager/Tmr_20mS/codegen/Task_20mS/Rx_Handler/ProcessMB11/Red_Mode_Cmd ==
  Input : Inport
  Action Port : ActionPort  ActionPortLabel=if(u1 == 1)
  Data Store Write1 : DataStoreWrite  DataStoreName=u8RedunModeCmd  IndexOptions=Index vector (dialog)  Indices=1  OutputSizes=1
  wires:
  Input/1 -> Data Store Write1/1

== system main/Task_Manager/Tmr_20mS/codegen/Task_20mS/Rx_Handler/ProcessMB12/Debug_Cmd ==
  Action Port : ActionPort  ActionPortLabel=elseif( u1==2)
  Constant3 : Constant  Value=[1:1]
  Data Store Read1 : DataStoreRead  DataStoreName=u8CanDataRx12  IndexOptions=Index vector (dialog)  Indices=1  OutputSizes=1
  Debug En/Dis : Subsystem  TreatAsAtomicUnit=on
  If1 : If  IfExpression=u1 == hex2dec('0xDA')  ElseIfExpressions=u1 == hex2dec('0xDB')
  Open Loop En Dis : Subsystem  TreatAsAtomicUnit=on
  Selector3 : Selector  IndexMode=Zero-based  InputPortWidth=8  IndexOptions=Index vector (port)  Indices=[1 3]  OutputSizes=1
  wires:
  Selector3/1 -> If1/1
  Constant3/1 -> Selector3/2
  Data Store Read1/1 -> Selector3/1
  If1/1 -> Debug En/Dis/Action
  If1/2 -> Open Loop En Dis/Action

== system main/Task_Manager/Tmr_20mS/codegen/Task_20mS/Rx_Handler/ProcessMB12/Debug_Read ==
  Action Port : ActionPort  ActionPortLabel=if(u1 == 0)
  Constant2 : Constant  Value=[1:1]
  Data Store Read : DataStoreRead  DataStoreName=u8CanDataRx12  IndexOptions=Index vector (dialog)  Indices=1  OutputSizes=1
  Debug_Cmd : Subsystem  TreatAsAtomicUnit=on
  Equal{,1..3} (4 alike) : RelationalOperator  Operator===  OutDataTypeStr=boolean  RndMeth=Simplest  InputSameDT=off
  If : If  IfExpression=u1 == 1
  OR : Logic  Operator=OR  Inputs=4  IconShape=distinctive  AllPortsSameDT=off  OutDataTypeStr=boolean
  RdReq_Calib : Constant  Value=0xD0
  RdReq_Deb1 : Constant  Value=0xD1
  RdReq_Deb2 : Constant  Value=0xD2
  RdReq_FwRev : Constant  Value=0xF0
  Selector1 : Selector  IndexMode=Zero-based  InputPortWidth=8  IndexOptions=Index vector (port)  Indices=[1 3]  OutputSizes=1
  wires:
  Constant2/1 -> Selector1/2
  Data Store Read/1 -> Selector1/1
  RdReq_FwRev/1 -> Equal/2
  RdReq_Calib/1 -> Equal1/2
  Selector1/1 -> Equal1/1, Equal2/1, Debug_Cmd/1(Input), Equal3/1, Equal/1
  RdReq_Deb2/1 -> Equal3/2
  RdReq_Deb1/1 -> Equal2/2
  Equal2/1 -> OR/3
  Equal3/1 -> OR/4
  Equal1/1 -> OR/2
  Equal/1 -> OR/1
  OR/1 -> If/1
  If/1 -> Debug_Cmd/Action

== system main/Task_Manager/Tmr_20mS/codegen/Task_20mS/Rx_Handler/ProcessMB12/Debug_Write ==
  Action Port : ActionPort  ActionPortLabel=elseif(u1 ==1)

== system main/Task_Manager/Tmr_20mS/codegen/Task_20mS/Tx_Handler/Run Tx Routine/TxReadRequest ==
  Action Port : ActionPort  ActionPortLabel=if(u1 == 1 & u2 == 1)
  Constant1 : Constant  Value=0  OutDataTypeStr=boolean
  Data Store Read2 : DataStoreRead  DataStoreName=u8RdReqMsgPntr  IndexOptions=Index vector (dialog)  Indices=1  OutputSizes=1
  Data Store Write1 : DataStoreWrite  DataStoreName=b01_ReadRequest  IndexOptions=Index vector (dialog)  Indices=1  OutputSizes=1
  Switch Case : SwitchCase  CaseConditions={0xF0, 0xD0, 0xD1, 0xD2}  ShowDefaultCase=off
  Tx Cal Data ID145 : Subsystem  TreatAsAtomicUnit=on
  Tx FW Rev ID144 : Subsystem  TreatAsAtomicUnit=on
  Tx TxDeb Dat1 146 : Subsystem  TreatAsAtomicUnit=on
  Tx TxDeb Dat2 147 : Subsystem  TreatAsAtomicUnit=on
  wires:
  Data Store Read2/1 -> Switch Case/1
  Switch Case/1 -> Tx FW Rev ID144/Action
  Switch Case/2 -> Tx Cal Data ID145/Action
  Switch Case/3 -> Tx TxDeb Dat1 146/Action
  Switch Case/4 -> Tx TxDeb Dat2 147/Action
  Constant1/1 -> Data Store Write1/1

== system main/Task_Manager/Tmr_20mS/codegen/Task_20mS/Tx_Handler/Run Tx Routine/TxStatusData ==
  Action Port : ActionPort  ActionPortLabel=else
  Data Store Read2 : DataStoreRead  DataStoreName=u8CanTxIndex  IndexOptions=Index vector (dialog)  Indices=1  OutputSizes=1
  Switch Case : SwitchCase  CaseConditions={0, 1, 2, 3, 4}  ShowDefaultCase=off
  Tx Sec Status ID120 : Subsystem  TreatAsAtomicUnit=on
  Tx Sec1 ID140 : Subsystem  TreatAsAtomicUnit=on
  Tx Sec2 ID141 : Subsystem  TreatAsAtomicUnit=on
  Tx Sec3 ID142 : Subsystem  TreatAsAtomicUnit=on
  Tx Sec4 ID143 : Subsystem  TreatAsAtomicUnit=on
  wires:
  Data Store Read2/1 -> Switch Case/1
  Switch Case/1 -> Tx Sec Status ID120/Action
  Switch Case/2 -> Tx Sec1 ID140/Action
  Switch Case/3 -> Tx Sec2 ID141/Action
  Switch Case/4 -> Tx Sec3 ID142/Action
  Switch Case/5 -> Tx Sec4 ID143/Action

== system main/Task_Manager/idle/idle_task/comm_npc/comm_npc/COMM_NPC.calcScixmtChksum/calc_chksum/For Iterator Subsystem ==
  scixmt_buffer : Inport
  Bitwise XOR : simulink/Logic and Bit Operations/Bitwise Operator  logicop=XOR  UseBitMask=off  NumInputPorts=2  BitMask=bin2dec('11011001')  BitMaskRealWorld=Stored Integer
  Data Store Read1 : DataStoreRead  DataStoreName=scixmt_chksum  IndexOptions=Index vector (dialog)  Indices=1  OutputSizes=1
  Data Store Write : DataStoreWrite  DataStoreName=scixmt_chksum  IndexOptions=Index vector (dialog)  Indices=1  OutputSizes=1
  For Iterator : ForIterator  IterationLimit=9  IndexMode=Zero-based  IterationVariableDataType=uint8
  Selector : Selector  IndexMode=Zero-based  InputPortWidth=12  IndexOptions=Index vector (port)  Indices=[1 3]  OutputSizes=1
  wires:
  For Iterator/1 -> Selector/2
  scixmt_buffer/1 -> Selector/1
  Selector/1 -> Bitwise XOR/1
  Bitwise XOR/1 -> Data Store Write/1
  Data Store Read1/1 -> Bitwise XOR/2

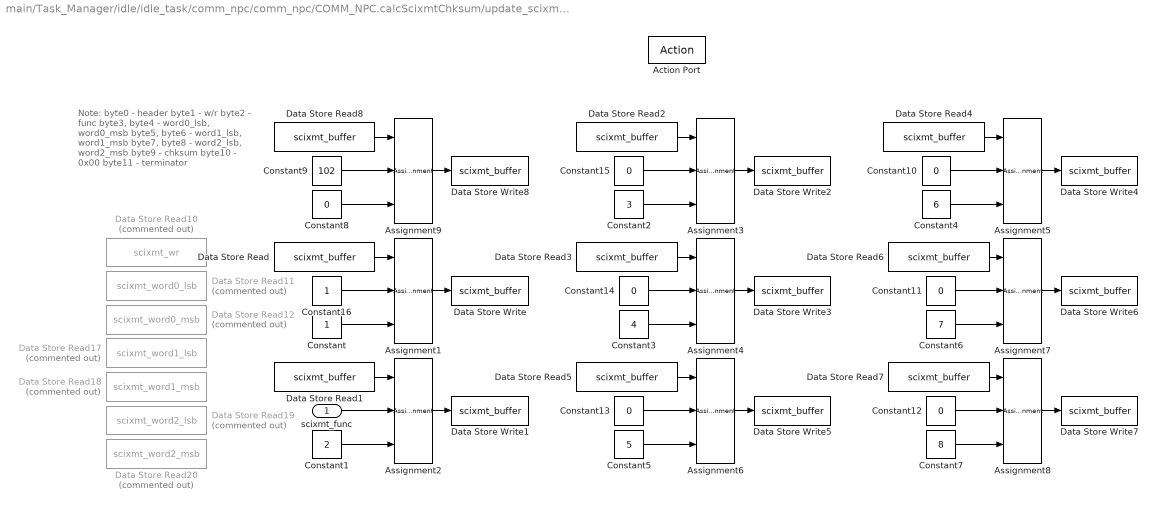
== system main/Task_Manager/idle/idle_task/comm_npc/comm_npc/COMM_NPC.calcScixmtChksum/update_scixmt_buffer/default ==
  note: Note:
      | byte0 - header
      | byte1 - w/r
      | byte2 - func
      | byte3, byte4 - word0_lsb, word0_msb
      | byte5, byte6 - word1_lsb, word1_msb
      | byte7, byte8 - word2_lsb, word2_msb
      | byte9 - chksum
      | byte10 - 0x00
      | byte11 - terminator
  scixmt_func : Inport
  Action Port : ActionPort  ActionPortLabel=else
  Assignment{1..9} (9 alike) : Assignment  IndexMode=Zero-based  DiagnosticForDimensions=Warning  IndexOptions=Index vector (port)  Indices=1  OutputSizes=1
  Constant : Constant  OutDataTypeStr=uint8
  Constant1 : Constant  Value=2  OutDataTypeStr=uint8
  Constant{8,10..15} (7 alike) : Constant  Value=0  OutDataTypeStr=uint8
  Constant16 : Constant  OutDataTypeStr=uint8
  Constant2 : Constant  Value=3  OutDataTypeStr=uint8
  Constant3 : Constant  Value=4  OutDataTypeStr=uint8
  Constant4 : Constant  Value=6  OutDataTypeStr=uint8
  Constant5 : Constant  Value=5  OutDataTypeStr=uint8
  Constant6 : Constant  Value=7  OutDataTypeStr=uint8
  Constant7 : Constant  Value=8  OutDataTypeStr=uint8
  Constant9 : Constant  Value=102  OutDataTypeStr=uint8
  Data Store Read{,1..8} (9 alike) : DataStoreRead  DataStoreName=scixmt_buffer  IndexOptions=Index vector (dialog)  Indices=1  OutputSizes=1
  Data Store Read10 : DataStoreRead  Commented=on  DataStoreName=scixmt_wr  IndexOptions=Index vector (dialog)  Indices=1  OutputSizes=1
  Data Store Read11 : DataStoreRead  Commented=on  DataStoreName=scixmt_word0_lsb  IndexOptions=Index vector (dialog)  Indices=1  OutputSizes=1
  Data Store Read12 : DataStoreRead  Commented=on  DataStoreName=scixmt_word0_msb  IndexOptions=Index vector (dialog)  Indices=1  OutputSizes=1
  Data Store Read17 : DataStoreRead  Commented=on  DataStoreName=scixmt_word1_lsb  IndexOptions=Index vector (dialog)  Indices=1  OutputSizes=1
  Data Store Read18 : DataStoreRead  Commented=on  DataStoreName=scixmt_word1_msb  IndexOptions=Index vector (dialog)  Indices=1  OutputSizes=1
  Data Store Read19 : DataStoreRead  Commented=on  DataStoreName=scixmt_word2_lsb  IndexOptions=Index vector (dialog)  Indices=1  OutputSizes=1
  Data Store Read20 : DataStoreRead  Commented=on  DataStoreName=scixmt_word2_msb  IndexOptions=Index vector (dialog)  Indices=1  OutputSizes=1
  Data Store Write{,1..8} (9 alike) : DataStoreWrite  DataStoreName=scixmt_buffer  IndexOptions=Index vector (dialog)  Indices=1  OutputSizes=1
  wires:
  scixmt_func/1 -> Assignment2/2
  Constant13/1 -> Assignment6/2
  Assignment1/1 -> Data Store Write/1
  Constant9/1 -> Assignment9/2
  Data Store Read8/1 -> Assignment9/1
  Assignment5/1 -> Data Store Write4/1
  Assignment9/1 -> Data Store Write8/1
  Constant11/1 -> Assignment7/2
  Constant/1 -> Assignment1/3
  Assignment6/1 -> Data Store Write5/1
  Constant2/1 -> Assignment3/3
  Constant5/1 -> Assignment6/3
  Data Store Read5/1 -> Assignment6/1
  Data Store Read7/1 -> Assignment8/1
  Constant4/1 -> Assignment5/3
  Data Store Read6/1 -> Assignment7/1
  Constant6/1 -> Assignment7/3
  Data Store Read1/1 -> Assignment2/1
  Assignment7/1 -> Data Store Write6/1
  Data Store Read4/1 -> Assignment5/1
  Constant7/1 -> Assignment8/3
  Data Store Read3/1 -> Assignment4/1
  Assignment8/1 -> Data Store Write7/1
  Data Store Read2/1 -> Assignment3/1
  Constant12/1 -> Assignment8/2
  Data Store Read/1 -> Assignment1/1
  Constant3/1 -> Assignment4/3
  Assignment3/1 -> Data Store Write2/1
  Constant10/1 -> Assignment5/2
  Constant14/1 -> Assignment4/2
  Assignment4/1 -> Data Store Write3/1
  Constant15/1 -> Assignment3/2
  Constant1/1 -> Assignment2/3
  Constant8/1 -> Assignment9/3
  Assignment2/1 -> Data Store Write1/1
  Constant16/1 -> Assignment1/2

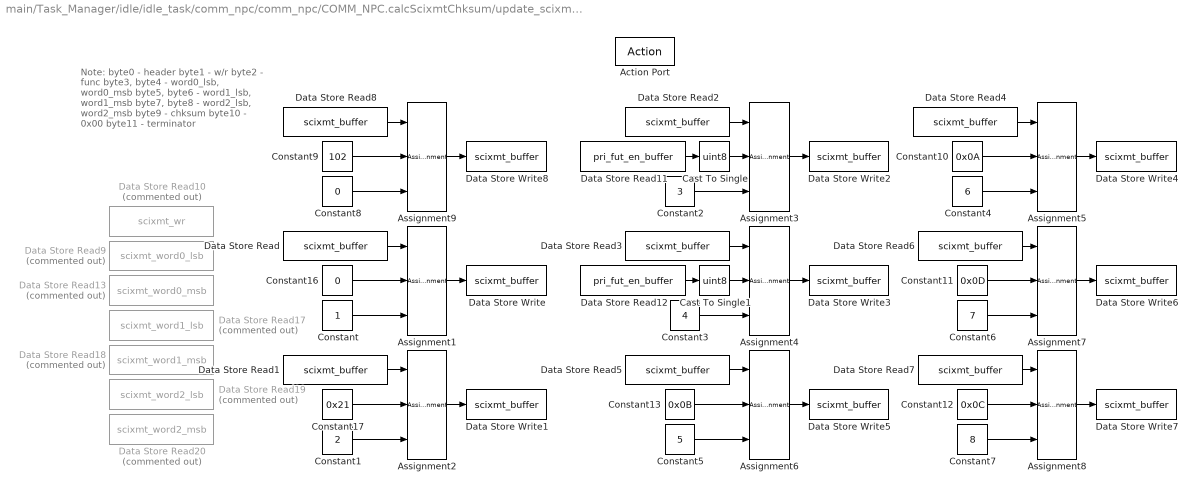
== system main/Task_Manager/idle/idle_task/comm_npc/comm_npc/COMM_NPC.calcScixmtChksum/update_scixmt_buffer/pri_fut_en ==
  note: Note:
      | byte0 - header
      | byte1 - w/r
      | byte2 - func
      | byte3, byte4 - word0_lsb, word0_msb
      | byte5, byte6 - word1_lsb, word1_msb
      | byte7, byte8 - word2_lsb, word2_msb
      | byte9 - chksum
      | byte10 - 0x00
      | byte11 - terminator
  Action Port : ActionPort  ActionPortLabel=if(u1 == 33)
  Assignment{1..9} (9 alike) : Assignment  IndexMode=Zero-based  DiagnosticForDimensions=Warning  IndexOptions=Index vector (port)  Indices=1  OutputSizes=1
  Cast To Single : DataTypeConversion  OutDataTypeStr=uint8  SaturateOnIntegerOverflow=off  RndMeth=Floor
  Cast To Single1 : DataTypeConversion  OutDataTypeStr=uint8  SaturateOnIntegerOverflow=off  RndMeth=Floor
  Constant : Constant  OutDataTypeStr=uint8
  Constant1 : Constant  Value=2  OutDataTypeStr=uint8
  Constant10 : Constant  Value=0x0A  OutDataTypeStr=uint8
  Constant11 : Constant  Value=0x0D  OutDataTypeStr=uint8
  Constant12 : Constant  Value=0x0C  OutDataTypeStr=uint8
  Constant13 : Constant  Value=0x0B  OutDataTypeStr=uint8
  Constant16 : Constant  Value=0  OutDataTypeStr=uint8
  Constant17 : Constant  Value=0x21  OutDataTypeStr=uint8
  Constant2 : Constant  Value=3  OutDataTypeStr=uint8
  Constant3 : Constant  Value=4  OutDataTypeStr=uint8
  Constant4 : Constant  Value=6  OutDataTypeStr=uint8
  Constant5 : Constant  Value=5  OutDataTypeStr=uint8
  Constant6 : Constant  Value=7  OutDataTypeStr=uint8
  Constant7 : Constant  Value=8  OutDataTypeStr=uint8
  Constant8 : Constant  Value=0  OutDataTypeStr=uint8
  Constant9 : Constant  Value=102  OutDataTypeStr=uint8
  Data Store Read{,1..8} (9 alike) : DataStoreRead  DataStoreName=scixmt_buffer  IndexOptions=Index vector (dialog)  Indices=1  OutputSizes=1
  Data Store Read10 : DataStoreRead  Commented=on  DataStoreName=scixmt_wr  IndexOptions=Index vector (dialog)  Indices=1  OutputSizes=1
  Data Store Read11 : DataStoreRead  DataStoreName=pri_fut_en_buffer  IndexOptions=Index vector (dialog)  Indices=1  OutputSizes=1
  Data Store Read12 : DataStoreRead  DataStoreName=pri_fut_en_buffer  IndexOptions=Index vector (dialog)  Indices=1  OutputSizes=1
  Data Store Read13 : DataStoreRead  Commented=on  DataStoreName=scixmt_word0_msb  IndexOptions=Index vector (dialog)  Indices=1  OutputSizes=1
  Data Store Read17 : DataStoreRead  Commented=on  DataStoreName=scixmt_word1_lsb  IndexOptions=Index vector (dialog)  Indices=1  OutputSizes=1
  Data Store Read18 : DataStoreRead  Commented=on  DataStoreName=scixmt_word1_msb  IndexOptions=Index vector (dialog)  Indices=1  OutputSizes=1
  Data Store Read19 : DataStoreRead  Commented=on  DataStoreName=scixmt_word2_lsb  IndexOptions=Index vector (dialog)  Indices=1  OutputSizes=1
  Data Store Read20 : DataStoreRead  Commented=on  DataStoreName=scixmt_word2_msb  IndexOptions=Index vector (dialog)  Indices=1  OutputSizes=1
  Data Store Read9 : DataStoreRead  Commented=on  DataStoreName=scixmt_word0_lsb  IndexOptions=Index vector (dialog)  Indices=1  OutputSizes=1
  Data Store Write{,1..8} (9 alike) : DataStoreWrite  DataStoreName=scixmt_buffer  IndexOptions=Index vector (dialog)  Indices=1  OutputSizes=1
  wires:
  Constant5/1 -> Assignment6/3
  Constant2/1 -> Assignment3/3
  Assignment9/1 -> Data Store Write8/1
  Constant11/1 -> Assignment7/2
  Assignment6/1 -> Data Store Write5/1
  Constant/1 -> Assignment1/3
  Data Store Read8/1 -> Assignment9/1
  Assignment1/1 -> Data Store Write/1
  Constant13/1 -> Assignment6/2
  Constant9/1 -> Assignment9/2
  Data Store Read2/1 -> Assignment3/1
  Constant17/1 -> Assignment2/2
  Assignment8/1 -> Data Store Write7/1
  Data Store Read/1 -> Assignment1/1
  Data Store Read3/1 -> Assignment4/1
  Constant12/1 -> Assignment8/2
  Data Store Read4/1 -> Assignment5/1
  Assignment7/1 -> Data Store Write6/1
  Constant7/1 -> Assignment8/3
  Constant6/1 -> Assignment7/3
  Data Store Read1/1 -> Assignment2/1
  Data Store Read5/1 -> Assignment6/1
  Data Store Read6/1 -> Assignment7/1
  Constant4/1 -> Assignment5/3
  Data Store Read7/1 -> Assignment8/1
  Constant16/1 -> Assignment1/2
  Constant1/1 -> Assignment2/3
  Constant10/1 -> Assignment5/2
  Constant8/1 -> Assignment9/3
  Assignment5/1 -> Data Store Write4/1
  Assignment2/1 -> Data Store Write1/1
  Constant3/1 -> Assignment4/3
  Assignment3/1 -> Data Store Write2/1
  Assignment4/1 -> Data Store Write3/1
  Data Store Read11/1 -> Cast To Single/1
  Cast To Single/1 -> Assignment3/2
  Cast To Single1/1 -> Assignment4/2
  Data Store Read12/1 -> Cast To Single1/1

== system main/Task_Manager/idle/idle_task/comm_npc/comm_npc/COMM_NPC.parseScircv/For Iterator Subsystem/header_found_before_bit13 ==
  scircv_buffer_tmp_idx0 : Inport
  Action Port : ActionPort  ActionPortLabel=if((u1 == 102) & (u2 < 13))
  Function-Call Generator1 : simulink/Ports & Subsystems/Function-Call Generator  sample_time=-1  numberOfIterations=1  DisallowWideOutput=off
  Function-Call Split1 : FunctionCallSplit  NumOutputPorts=2
  Function-Call Split4 : FunctionCallSplit  NumOutputPorts=2
  copy_to_scixmt_buffer : Subsystem  TreatAsAtomicUnit=on
  scircv_parse_ok : Subsystem  TreatAsAtomicUnit=on
  update_scircv_buffer_tmp_idx0 : Subsystem  TreatAsAtomicUnit=on
  Out1 : Outport  InitialOutput=[0]
  wires:
  Function-Call Split4/2 -> Function-Call Split1/1
  Function-Call Generator1/1 -> Function-Call Split4/1
  Function-Call Split4/1 -> update_scircv_buffer_tmp_idx0/Trigger
  scircv_buffer_tmp_idx0/1 -> update_scircv_buffer_tmp_idx0/1(Inport)
  Function-Call Split1/1 -> copy_to_scixmt_buffer/Trigger
  Function-Call Split1/2 -> scircv_parse_ok/Trigger
  scircv_parse_ok/1(Out1) -> Out1/1
